simulink model "xDamper"  (R2024b)
settings: Solver=FixedStepAuto  StartTime=0.0  StopTime=10.0  RelTol=1e-3  EnableMultiTasking=on
undefined symbols (not defined in the file): xDamperPotFLGain, xDamperPotFRGain, xDamperPotRLGain, xDamperPotRRGain
settings Model: DataDictionary=Master_Dictionary.sldd  EnableAccessToBaseWorkspace=off  Creator=torni  LastModifiedBy=Will
settings OptimizationCC: DefaultParameterBehavior=Inlined  EnhancedBackFolding=on  PassReuseOutputArgsAs=Individual arguments  ZeroExternalMemoryAtStartup=off  ZeroInternalMemoryAtStartup=off  MaxStackSize=8192  OptimizeBlockOrder=speed  DifferentSizesBufferReuse=on  OptimizationCustomize=off  EfficientTunableParamExpr=on
settings DebuggingCC: ParameterTunabilityLossMsg=error
settings HardwareCC: ProdBitPerPointer=32  ProdBitPerSizeT=32  ProdBitPerPtrDiffT=32  ProdLargestAtomicInteger=Long  ProdLargestAtomicFloat=Double  ProdWordSize=32  ProdLongLongMode=on  ProdHWDeviceType=ARM Compatible->ARM Cortex-M
settings SFSimCC: MATLABDynamicMemAlloc=off
settings RTWCC: Description=Embedded Coder  SystemTargetFile=ert.tlc  HardwareBoard=STM32H7xx Based (Single-core)  TemplateMakefile=ert_default_tmf  Toolchain=GNU Tools for ARM Embedded Processors
settings CodeAppCC: ForceParamTrailComments=on  IgnoreCustomStorageClasses=off  OperatorAnnotations=on  SimulinkDataObjDesc=on  SFDataObjDesc=on  InsertBlockDesc=on
settings ERTTargetCC: TargetLangStandard=C99 (ISO)  CodeReplacementLibrary=ARM Cortex-M  ExtModeTransport=3  ExtModeStaticAlloc=on  ExtModeStaticAllocSize=2048  ExtModeMexFile=ext_xcp  ExtModeIntrfLevel=Level2 - Open

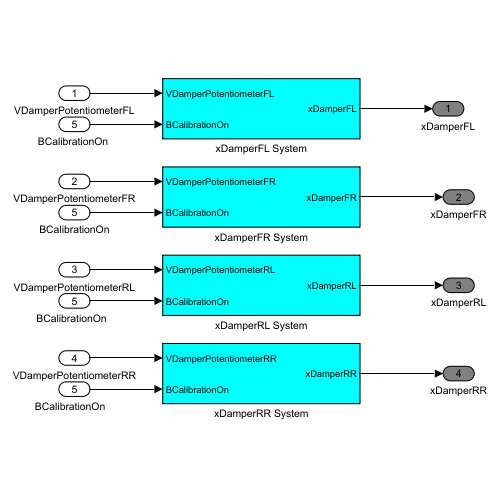
[thumbnail: Simulink's stored preview of the top-level diagram]
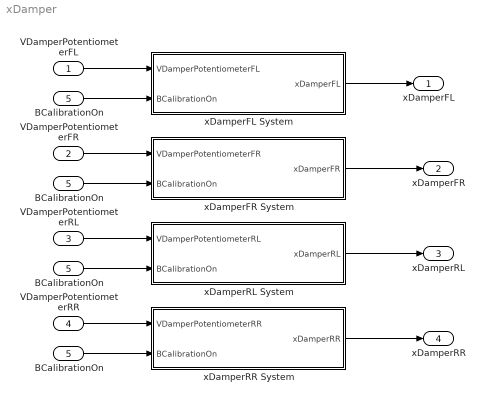
== system xDamper ==
  VDamperPotentiometerFL : Inport  OutDataTypeStr=double
  "VDamperPotentiometerFR " : Inport  Port=2  OutDataTypeStr=double
  VDamperPotentiometerRL : Inport  Port=3  OutDataTypeStr=double
  VDamperPotentiometerRR : Inport  Port=4  OutDataTypeStr=double
  BCalibrationOn : Inport  Port=5  OutDataTypeStr=boolean
  "BCalibrationOn " : InportShadow  Port=5  OutDataTypeStr=boolean
  "BCalibrationOn  " : InportShadow  Port=5  OutDataTypeStr=boolean
  "BCalibrationOn   " : InportShadow  Port=5  OutDataTypeStr=boolean
  xDamperFL System : Subsystem
  xDamperFR System : Subsystem
  xDamperRL System : Subsystem
  xDamperRR System : Subsystem
  xDamperFL : Outport  OutDataTypeStr=double  VectorParamsAs1DForOutWhenUnconnected=off
  xDamperFR : Outport  Port=2  OutDataTypeStr=double  VectorParamsAs1DForOutWhenUnconnected=off
  xDamperRL : Outport  Port=3  OutDataTypeStr=double  VectorParamsAs1DForOutWhenUnconnected=off
  xDamperRR : Outport  Port=4  OutDataTypeStr=double  VectorParamsAs1DForOutWhenUnconnected=off
  wires:
  VDamperPotentiometerFL/1 -> xDamperFL System/1(VDamperPotentiometerFL)
  BCalibrationOn/1 -> xDamperFR System/2(BCalibrationOn)
  "VDamperPotentiometerFR "/1 -> xDamperFR System/1(VDamperPotentiometerFR)
  xDamperFR System/1(xDamperFR) -> xDamperFR/1
  xDamperFL System/1(xDamperFL) -> xDamperFL/1
  "BCalibrationOn "/1 -> xDamperFL System/2(BCalibrationOn)
  VDamperPotentiometerRL/1 -> xDamperRL System/1(VDamperPotentiometerRL)
  xDamperRL System/1(xDamperRL) -> xDamperRL/1
  "BCalibrationOn  "/1 -> xDamperRL System/2(BCalibrationOn)
  VDamperPotentiometerRR/1 -> xDamperRR System/1(VDamperPotentiometerRR)
  xDamperRR System/1(xDamperRR) -> xDamperRR/1
  "BCalibrationOn   "/1 -> xDamperRR System/2(BCalibrationOn)

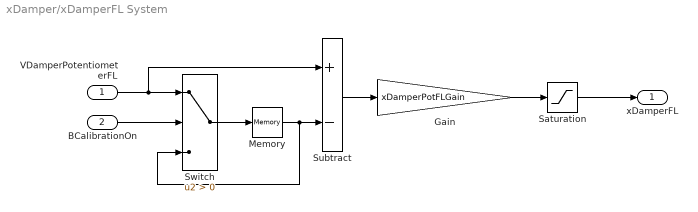
== system xDamper/xDamperFL System ==
  VDamperPotentiometerFL : Inport  OutDataTypeStr=double
  BCalibrationOn : Inport  Port=2  OutDataTypeStr=boolean
  Gain : Gain  Gain=xDamperPotFLGain
  Memory : Memory  InitialCondition=500  InheritSampleTime=on
  Saturation : Saturate  UpperLimit=150  LowerLimit=-50
  Subtract : Sum  Inputs=+-
  Switch : Switch  Criteria=u2 > Threshold  SaturateOnIntegerOverflow=off  InputSameDT=off
  xDamperFL : Outport  VectorParamsAs1DForOutWhenUnconnected=off
  wires:
  Saturation/1 -> xDamperFL/1
  Gain/1 -> Saturation/1
  Subtract/1 -> Gain/1
  Memory/1 -> Subtract/2, Switch/3
  Switch/1 -> Memory/1
  BCalibrationOn/1 -> Switch/2
  VDamperPotentiometerFL/1 -> Switch/1, Subtract/1

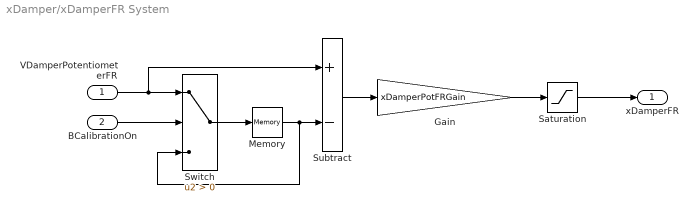
== system xDamper/xDamperFR System ==
  VDamperPotentiometerFR : Inport  OutDataTypeStr=double
  BCalibrationOn : Inport  Port=2  OutDataTypeStr=boolean
  Gain : Gain  Gain=xDamperPotFRGain
  Memory : Memory  InitialCondition=500  InheritSampleTime=on
  Saturation : Saturate  UpperLimit=150  LowerLimit=-50
  Subtract : Sum  Inputs=+-
  Switch : Switch  Criteria=u2 > Threshold  SaturateOnIntegerOverflow=off  InputSameDT=off
  xDamperFR : Outport  VectorParamsAs1DForOutWhenUnconnected=off
  wires:
  VDamperPotentiometerFR/1 -> Subtract/1, Switch/1
  BCalibrationOn/1 -> Switch/2
  Switch/1 -> Memory/1
  Memory/1 -> Switch/3, Subtract/2
  Subtract/1 -> Gain/1
  Gain/1 -> Saturation/1
  Saturation/1 -> xDamperFR/1

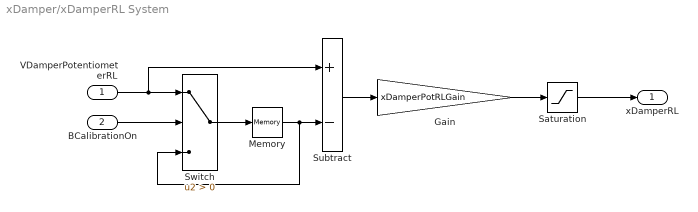
== system xDamper/xDamperRL System ==
  VDamperPotentiometerRL : Inport  OutDataTypeStr=double
  BCalibrationOn : Inport  Port=2  OutDataTypeStr=boolean
  Gain : Gain  Gain=xDamperPotRLGain
  Memory : Memory  InitialCondition=500  InheritSampleTime=on
  Saturation : Saturate  UpperLimit=150  LowerLimit=-50
  Subtract : Sum  Inputs=+-
  Switch : Switch  Criteria=u2 > Threshold  SaturateOnIntegerOverflow=off  InputSameDT=off
  xDamperRL : Outport  VectorParamsAs1DForOutWhenUnconnected=off
  wires:
  VDamperPotentiometerRL/1 -> Subtract/1, Switch/1
  BCalibrationOn/1 -> Switch/2
  Switch/1 -> Memory/1
  Memory/1 -> Switch/3, Subtract/2
  Subtract/1 -> Gain/1
  Gain/1 -> Saturation/1
  Saturation/1 -> xDamperRL/1

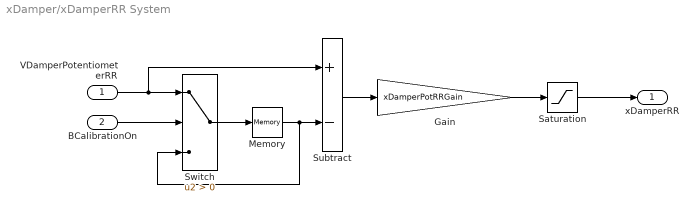
== system xDamper/xDamperRR System ==
  VDamperPotentiometerRR : Inport  OutDataTypeStr=double
  BCalibrationOn : Inport  Port=2  OutDataTypeStr=boolean
  Gain : Gain  Gain=xDamperPotRRGain
  Memory : Memory  InitialCondition=500  InheritSampleTime=on
  Saturation : Saturate  UpperLimit=150  LowerLimit=-50
  Subtract : Sum  Inputs=+-
  Switch : Switch  Criteria=u2 > Threshold  SaturateOnIntegerOverflow=off  InputSameDT=off
  xDamperRR : Outport  VectorParamsAs1DForOutWhenUnconnected=off
  wires:
  Saturation/1 -> xDamperRR/1
  Gain/1 -> Saturation/1
  Subtract/1 -> Gain/1
  Memory/1 -> Subtract/2, Switch/3
  Switch/1 -> Memory/1
  BCalibrationOn/1 -> Switch/2
  VDamperPotentiometerRR/1 -> Switch/1, Subtract/1
